simulink library "gnss_sdr_galileo_e1_tcp_connector_tracking_lib"  (Simulink 7.6)
settings: Solver=VariableStepDiscrete  StartTime=0.0  StopTime=10.0  RelTol=1e-3
undefined symbols (not defined in the file or in its folder): B_DLL, B_PLL, d_pdi_carr, d_pdi_code, k_DLL, k_PLL, magnitude, zeta_DLL, zeta_PLL
libraries: simulink x746, instrumentlib x2, dspindex x1
(part 1 of 5)
settings Model: Creator=David Pubill  LastModifiedBy=David Pubill

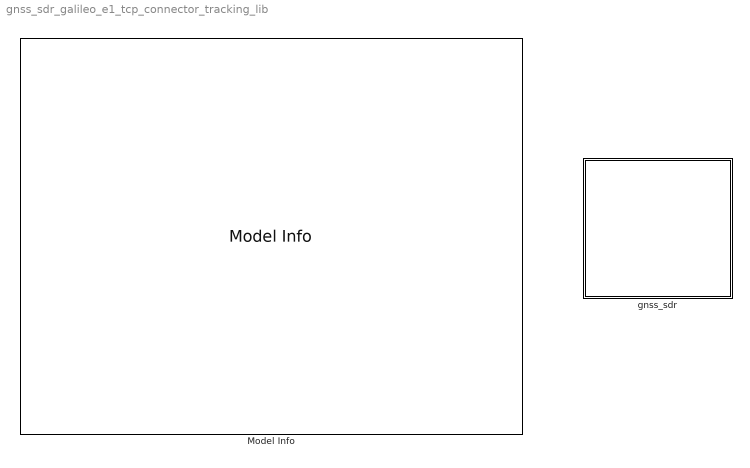
== system gnss_sdr_galileo_e1_tcp_connector_tracking_lib ==
  Model Info : simulink/Model-Wide Utilities/Model Info  SystemSampleTime=-1  InitialBlockCM=None  BlockCM=None  Frame=on  DisplayStringWithTags=|  HorizontalTextAlignment=Left  LeftAlignmentValue=0.02  SourceBlockDiagram=gnss_sdr_galileo_e1_tcp_connector_tracking_lib  TagMaxNumber=20
      | /*! 
      |   * \file gnss_sdr_galileo_e1_tcp_connector_tracking_lib.mdl
      |   * \brief  gnss_sdr_galileo_e1_tcp_connector_tracking Simulink library model. For 
      |   * further information, please check  the README_gnss_sdr_galileo_e1_tcp_connector_tracking.txt file.
      |   *
      |   * \author David Pubill, 2012. dpubill(at)cttc.es
      |   * -------------------------------------------------------------------------
      |   *
      |   * Copyright (C) 2010-2012  (see AUTHORS file for a list of contributors)
      |   *
      |   * GNSS-SDR is a software defined Global Navigation
      |   *          Satellite Systems receiver
      |   *
      |   * This file is part of GNSS-SDR.
      |   *
      |   * GNSS-SDR is free software: you can redistribute it and/or modify
      |   * it under the terms of the GNU General Public License as published by
      |   * the Free Software Foundation, either version 3 of the License, or
      |   * at your option) any later version.
      |   *
      |   * GNSS-SDR is distributed in the hope that it will be useful,
      |   * but WITHOUT ANY WARRANTY; without even the implied warranty of
      |   * MERCHANTABILITY or FITNESS FOR A PARTICULAR PURPOSE.  See the
      |   * GNU General Public License for more details.
      |   *
      |   * You should have received a copy of the GNU General Public License
      |   * along with GNSS-SDR. If not, see <http://www.gnu.org/licenses/>.
      |   *
      |   * -------------------------------------------------------------------------
      |   */
  gnss_sdr : Subsystem

== system gnss_sdr_galileo_e1_tcp_connector_tracking_lib/gnss_sdr ==
  gnss_sdr_galileo_e1_tcp_connector_tracking : Subsystem
  gnss_sdr_galileo_e1_tcp_connector_tracking_rx : Subsystem
  gnss_sdr_galileo_e1_tcp_connector_tracking_tx : Subsystem

== system gnss_sdr_galileo_e1_tcp_connector_tracking_lib/gnss_sdr/gnss_sdr_galileo_e1_tcp_connector_tracking ==
  control_id : Inport
  d_vE_I : Inport  Port=2
  d_vE_Q : Inport  Port=3
  d_E_I : Inport  Port=4
  d_E_Q : Inport  Port=5
  d_L_I : Inport  Port=6
  d_L_Q : Inport  Port=7
  d_vL_I : Inport  Port=8
  d_vL_Q : Inport  Port=9
  d_P_I : Inport  Port=10
  d_P_Q : Inport  Port=11
  d_acq_carrier_doppler_Hz : Inport  Port=12
  enable_tracking : Inport  Port=13
  Abs{,1..4} (5 alike) : Abs
  Carrier Tracking (PLL) : Subsystem
  Code Tracking (DLL) : Subsystem
  Data Type  Conversion1 : DataTypeConversion  OutDataTypeStr=single  SaturateOnIntegerOverflow=on  RndMeth=Zero
  Data Type  Conversion{2,5..9} (6 alike) : DataTypeConversion  OutDataTypeStr=double  SaturateOnIntegerOverflow=on  RndMeth=Zero
  Data Type  Conversion3 : DataTypeConversion  OutDataTypeStr=single  SaturateOnIntegerOverflow=on  RndMeth=Zero
  Data Type  Conversion4 : DataTypeConversion  OutDataTypeStr=single  SaturateOnIntegerOverflow=on  RndMeth=Zero
  Mux : Mux  Inputs=5
  Real-Imag to Complex{,1..4} (5 alike) : RealImagToComplex
  control_id_ : Outport
  code_nco : Outport  Port=2
  carr_nco : Outport  Port=3
  carrier_doppler_Hz : Outport  Port=4
  EPL Scope : Outport  Port=5
  wires:
  Data Type  Conversion8/1 -> Code Tracking (DLL)/4(vL), Abs3/1
  Data Type  Conversion7/1 -> Code Tracking (DLL)/1(vE), Abs4/1
  d_vL_Q/1 -> Real-Imag to Complex4/2
  d_vL_I/1 -> Real-Imag to Complex4/1
  Real-Imag to Complex4/1 -> Data Type  Conversion8/1
  d_vE_Q/1 -> Real-Imag to Complex3/2
  d_vE_I/1 -> Real-Imag to Complex3/1
  Real-Imag to Complex3/1 -> Data Type  Conversion7/1
  Mux/1 -> EPL Scope/1
  enable_tracking/1 -> Carrier Tracking (PLL)/3(enable_tracking), Code Tracking (DLL)/5(enable_tracking)
  Data Type  Conversion3/1 -> carrier_doppler_Hz/1
  d_acq_carrier_doppler_Hz/1 -> Data Type  Conversion9/1
  Data Type  Conversion6/1 -> Carrier Tracking (PLL)/1(P), Abs1/1
  Data Type  Conversion5/1 -> Abs/1, Code Tracking (DLL)/3(L)
  Data Type  Conversion2/1 -> Abs2/1, Code Tracking (DLL)/2(E)
  d_P_Q/1 -> Real-Imag to Complex2/2
  d_P_I/1 -> Real-Imag to Complex2/1
  d_L_Q/1 -> Real-Imag to Complex1/2
  d_L_I/1 -> Real-Imag to Complex1/1
  control_id/1 -> control_id_/1
  Data Type  Conversion4/1 -> carr_nco/1
  Data Type  Conversion1/1 -> code_nco/1
  d_E_Q/1 -> Real-Imag to Complex/2
  d_E_I/1 -> Real-Imag to Complex/1
  Real-Imag to Complex2/1 -> Data Type  Conversion6/1
  Real-Imag to Complex1/1 -> Data Type  Conversion5/1
  Carrier Tracking (PLL)/1(carr_nco) -> Data Type  Conversion4/1
  Real-Imag to Complex/1 -> Data Type  Conversion2/1
  Code Tracking (DLL)/1(code_nco) -> Data Type  Conversion1/1
  Carrier Tracking (PLL)/2(carrier_doppler_Hz) -> Data Type  Conversion3/1
  Abs4/1 -> Mux/1
  Abs2/1 -> Mux/2
  Abs1/1 -> Mux/3
  Abs/1 -> Mux/4
  Abs3/1 -> Mux/5
  Data Type  Conversion9/1 -> Carrier Tracking (PLL)/2(d_acq_carrier_doppler_Hz)

== system gnss_sdr_galileo_e1_tcp_connector_tracking_lib/gnss_sdr/gnss_sdr_galileo_e1_tcp_connector_tracking_rx ==
  Multiport Selector : dspindex/Multiport Selector  rowsOrCols=Rows  idxCellArray={1,2,3,4,5,6,7,8,9,10,11,12,13,14,15,16,17,18,19,20,21,22,23,24,25,26,27,28,29,30,31,32,33,34,35,36,37,38,39,40,41,42,43,44,45,46,47,48,49,50,51,52}  idxErrMode=Clip Index
  RX : instrumentlib/TCP//IP Receive  DialogController=instrumentcreatedialog  DialogControllerArgs=DataTag4  Host=84.88.61.86  Port=2070  DataSize=52  EnableBlockingMode=on  Timeout=5  SampleTime=-1  DataType=uint8  ByteOrder=BigEndian
  Subsystem : Subsystem
  Subsystem1 : Subsystem
  Subsystem10 : Subsystem  AncestorBlock=gnss_sdr_galileo_e1_tcp_connector_tracking_lib/gnss_sdr/gnss_sdr_galileo_e1_tcp_connector_tracking_rx/Subsystem1
  Subsystem11 : Subsystem  AncestorBlock=gnss_sdr_galileo_e1_tcp_connector_tracking_lib/gnss_sdr/gnss_sdr_galileo_e1_tcp_connector_tracking_rx/Subsystem2
  Subsystem12 : Subsystem  AncestorBlock=gnss_sdr_galileo_e1_tcp_connector_tracking_lib/gnss_sdr/gnss_sdr_galileo_e1_tcp_connector_tracking_rx/Subsystem3
  Subsystem2 : Subsystem
  Subsystem3 : Subsystem
  Subsystem4 : Subsystem
  Subsystem5 : Subsystem
  Subsystem6 : Subsystem
  Subsystem7 : Subsystem
  Subsystem8 : Subsystem
  Subsystem9 : Subsystem  AncestorBlock=gnss_sdr_galileo_e1_tcp_connector_tracking_lib/gnss_sdr/gnss_sdr_galileo_e1_tcp_connector_tracking_rx/Subsystem
  control_id : Outport
  d_vE_I : Outport  Port=2
  d_vE_Q : Outport  Port=3
  d_E_I : Outport  Port=4
  d_E_Q : Outport  Port=5
  d_L_I : Outport  Port=6
  d_L_Q : Outport  Port=7
  d_vL_I : Outport  Port=8
  d_vL_Q : Outport  Port=9
  d_P_I : Outport  Port=10
  d_P_Q : Outport  Port=11
  d_acq_carrier_doppler_Hz : Outport  Port=12
  enable_tracking : Outport  Port=13
  wires:
  Multiport Selector/52 -> Subsystem7/4(In4)
  Multiport Selector/51 -> Subsystem7/3(In3)
  Multiport Selector/50 -> Subsystem7/2(In2)
  Multiport Selector/49 -> Subsystem7/1(In1)
  Multiport Selector/48 -> Subsystem6/4(In4)
  Multiport Selector/47 -> Subsystem6/3(In3)
  Multiport Selector/46 -> Subsystem6/2(In2)
  Multiport Selector/45 -> Subsystem6/1(In1)
  Multiport Selector/44 -> Subsystem5/4(In4)
  Multiport Selector/43 -> Subsystem5/3(In3)
  Multiport Selector/42 -> Subsystem5/2(In2)
  Multiport Selector/41 -> Subsystem5/1(In1)
  Multiport Selector/40 -> Subsystem4/4(In4)
  Multiport Selector/39 -> Subsystem4/3(In3)
  Multiport Selector/38 -> Subsystem4/2(In2)
  Multiport Selector/37 -> Subsystem4/1(In1)
  Multiport Selector/36 -> Subsystem12/4(In4)
  Multiport Selector/35 -> Subsystem12/3(In3)
  Multiport Selector/34 -> Subsystem12/2(In2)
  Multiport Selector/33 -> Subsystem12/1(In1)
  Multiport Selector/32 -> Subsystem11/4(In4)
  Multiport Selector/31 -> Subsystem11/3(In3)
  Multiport Selector/30 -> Subsystem11/2(In2)
  Multiport Selector/29 -> Subsystem11/1(In1)
  Multiport Selector/28 -> Subsystem3/4(In4)
  Multiport Selector/27 -> Subsystem3/3(In3)
  Multiport Selector/26 -> Subsystem3/2(In2)
  Multiport Selector/25 -> Subsystem3/1(In1)
  Multiport Selector/24 -> Subsystem2/4(In4)
  Multiport Selector/23 -> Subsystem2/3(In3)
  Multiport Selector/22 -> Subsystem2/2(In2)
  Multiport Selector/21 -> Subsystem2/1(In1)
  Multiport Selector/20 -> Subsystem1/4(In4)
  Multiport Selector/19 -> Subsystem1/3(In3)
  Multiport Selector/18 -> Subsystem1/2(In2)
  Multiport Selector/17 -> Subsystem1/1(In1)
  Multiport Selector/16 -> Subsystem/4(In4)
  Multiport Selector/15 -> Subsystem/3(In3)
  Multiport Selector/14 -> Subsystem/2(In2)
  Multiport Selector/13 -> Subsystem/1(In1)
  Multiport Selector/12 -> Subsystem10/4(In4)
  Multiport Selector/11 -> Subsystem10/3(In3)
  Multiport Selector/10 -> Subsystem10/2(In2)
  Multiport Selector/9 -> Subsystem10/1(In1)
  Multiport Selector/8 -> Subsystem9/4(In4)
  Multiport Selector/7 -> Subsystem9/3(In3)
  Multiport Selector/6 -> Subsystem9/2(In2)
  Multiport Selector/5 -> Subsystem9/1(In1)
  Multiport Selector/4 -> Subsystem8/4(In4)
  Multiport Selector/3 -> Subsystem8/3(In3)
  Multiport Selector/2 -> Subsystem8/2(In2)
  Multiport Selector/1 -> Subsystem8/1(In1)
  Subsystem11/1(d_vL_I) -> d_vL_I/1
  Subsystem12/1(d_vL_Q) -> d_vL_Q/1
  Subsystem9/1(d_vE_I) -> d_vE_I/1
  Subsystem10/1(d_vE_Q) -> d_vE_Q/1
  Subsystem7/1(enable_tracking) -> enable_tracking/1
  Subsystem6/1(d_acq_carrier_doppler_Hz) -> d_acq_carrier_doppler_Hz/1
  Subsystem5/1(d_P_Q) -> d_P_Q/1
  Subsystem8/1(control_id) -> control_id/1
  Subsystem/1(d_E_I) -> d_E_I/1
  Subsystem1/1(d_E_Q) -> d_E_Q/1
  Subsystem2/1(d_L_I) -> d_L_I/1
  Subsystem3/1(d_L_Q) -> d_L_Q/1
  Subsystem4/1(d_P_I) -> d_P_I/1
  RX/1 -> Multiport Selector/1

== system gnss_sdr_galileo_e1_tcp_connector_tracking_lib/gnss_sdr/gnss_sdr_galileo_e1_tcp_connector_tracking_tx ==
  control_id : Inport
  code_nco : Inport  Port=2
  carr_nco : Inport  Port=3
  carrier_doppler_Hz : Inport  Port=4
  TX : instrumentlib/TCP//IP Send  DialogController=instrumentcreatedialog  DialogControllerArgs=DataTag5  Host=84.88.61.86  Port=2070  EnableBlockingMode=on  Timeout=5  ByteOrder=LittleEndian
  Vector Concatenate1 : Concatenate  NumInputs=4  Mode=Vector
  wires:
  carrier_doppler_Hz/1 -> Vector Concatenate1/4
  Vector Concatenate1/1 -> TX/1
  control_id/1 -> Vector Concatenate1/1
  code_nco/1 -> Vector Concatenate1/2
  carr_nco/1 -> Vector Concatenate1/3

== system gnss_sdr_galileo_e1_tcp_connector_tracking_lib/gnss_sdr/gnss_sdr_galileo_e1_tcp_connector_tracking/Carrier Tracking (PLL) ==
  P : Inport
  d_acq_carrier_doppler_Hz : Inport  Port=2
  enable_tracking : Inport  Port=3
  Constant : Constant  Value=0  SampleTime=-1
  PLL Filter : Subsystem
  PLL discriminator : Subsystem  AncestorBlock=|
      | gnss_sdr_tcp_connector_tracking_lib/gnss_sdr/gnss_sdr_tcp_connector_tracking/Carrier Tracking 
      | (PLL)/atan2(Q,I)1/PLL Costas loop two quadrant arctan discriminator
  Subtract : Sum
  Switch : Switch  Threshold=1
  "[rad/s] to [Hz]" : Gain  Gain=1/(2*pi)
  carr_nco : Outport
  carrier_doppler_Hz : Outport  Port=2
  wires:
  PLL discriminator/1(carr_error) -> "[rad/s] to [Hz]"/1
  P/1 -> PLL discriminator/1(P)
  enable_tracking/1 -> Switch/2, PLL Filter/2(enable_tracking)
  PLL Filter/1(carr_nco) -> Subtract/1, Switch/1
  d_acq_carrier_doppler_Hz/1 -> Subtract/2
  Subtract/1 -> carrier_doppler_Hz/1
  Switch/1 -> carr_nco/1
  Constant/1 -> Switch/3
  "[rad/s] to [Hz]"/1 -> PLL Filter/1(carr_error)

== system gnss_sdr_galileo_e1_tcp_connector_tracking_lib/gnss_sdr/gnss_sdr_galileo_e1_tcp_connector_tracking/Code Tracking (DLL) ==
  vE : Inport
  E : Inport  Port=2
  L : Inport  Port=3
  vL : Inport  Port=4
  enable_tracking : Inport  Port=5
  DLL Filter : Subsystem
  DLL discriminator : Subsystem
  code_nco : Outport
  wires:
  vL/1 -> DLL discriminator/4(vL)
  vE/1 -> DLL discriminator/1(vE)
  E/1 -> DLL discriminator/2(E)
  L/1 -> DLL discriminator/3(L)
  DLL Filter/1(code_nco) -> code_nco/1
  DLL discriminator/1(code_error) -> DLL Filter/1(code_error)
  enable_tracking/1 -> DLL Filter/2(enable_tracking)

== system gnss_sdr_galileo_e1_tcp_connector_tracking_lib/gnss_sdr/gnss_sdr_galileo_e1_tcp_connector_tracking_rx/Subsystem ==
  In1 : Inport
  In2 : Inport  Port=2
  In3 : Inport  Port=3
  In4 : Inport  Port=4
  Data Type  Conversion{1..5} (5 alike) : DataTypeConversion  OutDataTypeStr=single  SaturateOnIntegerOverflow=on  RndMeth=Zero
  hex2float : Subsystem
  d_E_I : Outport  OutputWhenDisabled=reset  InitialOutput=0
  wires:
  In1/1 -> Data Type  Conversion3/1
  In2/1 -> Data Type  Conversion2/1
  In3/1 -> Data Type  Conversion1/1
  In4/1 -> Data Type  Conversion4/1
  Data Type  Conversion3/1 -> hex2float/4(In4)
  Data Type  Conversion2/1 -> hex2float/3(In3)
  Data Type  Conversion1/1 -> hex2float/2(In2)
  Data Type  Conversion4/1 -> hex2float/1(In1)
  hex2float/1(Out1) -> Data Type  Conversion5/1
  Data Type  Conversion5/1 -> d_E_I/1

== system gnss_sdr_galileo_e1_tcp_connector_tracking_lib/gnss_sdr/gnss_sdr_galileo_e1_tcp_connector_tracking_rx/Subsystem1 ==
  In1 : Inport
  In2 : Inport  Port=2
  In3 : Inport  Port=3
  In4 : Inport  Port=4
  Data Type  Conversion{1..5} (5 alike) : DataTypeConversion  OutDataTypeStr=single  SaturateOnIntegerOverflow=on  RndMeth=Zero
  hex2float : Subsystem
  d_E_Q : Outport  OutputWhenDisabled=reset  InitialOutput=0
  wires:
  Data Type  Conversion5/1 -> d_E_Q/1
  hex2float/1(Out1) -> Data Type  Conversion5/1
  Data Type  Conversion4/1 -> hex2float/1(In1)
  Data Type  Conversion1/1 -> hex2float/2(In2)
  Data Type  Conversion2/1 -> hex2float/3(In3)
  Data Type  Conversion3/1 -> hex2float/4(In4)
  In4/1 -> Data Type  Conversion4/1
  In3/1 -> Data Type  Conversion1/1
  In2/1 -> Data Type  Conversion2/1
  In1/1 -> Data Type  Conversion3/1

== system gnss_sdr_galileo_e1_tcp_connector_tracking_lib/gnss_sdr/gnss_sdr_galileo_e1_tcp_connector_tracking_rx/Subsystem10 ==
  In1 : Inport
  In2 : Inport  Port=2
  In3 : Inport  Port=3
  In4 : Inport  Port=4
  Data Type  Conversion{1..5} (5 alike) : DataTypeConversion  OutDataTypeStr=single  SaturateOnIntegerOverflow=on  RndMeth=Zero
  hex2float : Subsystem
  d_vE_Q : Outport  OutputWhenDisabled=reset  InitialOutput=0
  wires:
  Data Type  Conversion5/1 -> d_vE_Q/1
  hex2float/1(Out1) -> Data Type  Conversion5/1
  Data Type  Conversion4/1 -> hex2float/1(In1)
  Data Type  Conversion1/1 -> hex2float/2(In2)
  Data Type  Conversion2/1 -> hex2float/3(In3)
  Data Type  Conversion3/1 -> hex2float/4(In4)
  In4/1 -> Data Type  Conversion4/1
  In3/1 -> Data Type  Conversion1/1
  In2/1 -> Data Type  Conversion2/1
  In1/1 -> Data Type  Conversion3/1

== system gnss_sdr_galileo_e1_tcp_connector_tracking_lib/gnss_sdr/gnss_sdr_galileo_e1_tcp_connector_tracking_rx/Subsystem11 ==
  In1 : Inport
  In2 : Inport  Port=2
  In3 : Inport  Port=3
  In4 : Inport  Port=4
  Data Type  Conversion{1..5} (5 alike) : DataTypeConversion  OutDataTypeStr=single  SaturateOnIntegerOverflow=on  RndMeth=Zero
  hex2float : Subsystem
  d_vL_I : Outport  OutputWhenDisabled=reset  InitialOutput=0
  wires:
  In1/1 -> Data Type  Conversion3/1
  In2/1 -> Data Type  Conversion2/1
  In3/1 -> Data Type  Conversion1/1
  In4/1 -> Data Type  Conversion4/1
  Data Type  Conversion3/1 -> hex2float/4(In4)
  Data Type  Conversion2/1 -> hex2float/3(In3)
  Data Type  Conversion1/1 -> hex2float/2(In2)
  Data Type  Conversion4/1 -> hex2float/1(In1)
  hex2float/1(Out1) -> Data Type  Conversion5/1
  Data Type  Conversion5/1 -> d_vL_I/1

== system gnss_sdr_galileo_e1_tcp_connector_tracking_lib/gnss_sdr/gnss_sdr_galileo_e1_tcp_connector_tracking_rx/Subsystem12 ==
  In1 : Inport
  In2 : Inport  Port=2
  In3 : Inport  Port=3
  In4 : Inport  Port=4
  Data Type  Conversion{1..5} (5 alike) : DataTypeConversion  OutDataTypeStr=single  SaturateOnIntegerOverflow=on  RndMeth=Zero
  hex2float : Subsystem
  d_vL_Q : Outport  OutputWhenDisabled=reset  InitialOutput=0
  wires:
  Data Type  Conversion5/1 -> d_vL_Q/1
  hex2float/1(Out1) -> Data Type  Conversion5/1
  Data Type  Conversion4/1 -> hex2float/1(In1)
  Data Type  Conversion1/1 -> hex2float/2(In2)
  Data Type  Conversion2/1 -> hex2float/3(In3)
  Data Type  Conversion3/1 -> hex2float/4(In4)
  In4/1 -> Data Type  Conversion4/1
  In3/1 -> Data Type  Conversion1/1
  In2/1 -> Data Type  Conversion2/1
  In1/1 -> Data Type  Conversion3/1

== system gnss_sdr_galileo_e1_tcp_connector_tracking_lib/gnss_sdr/gnss_sdr_galileo_e1_tcp_connector_tracking_rx/Subsystem2 ==
  In1 : Inport
  In2 : Inport  Port=2
  In3 : Inport  Port=3
  In4 : Inport  Port=4
  Data Type  Conversion{1..5} (5 alike) : DataTypeConversion  OutDataTypeStr=single  SaturateOnIntegerOverflow=on  RndMeth=Zero
  hex2float : Subsystem
  d_L_I : Outport  OutputWhenDisabled=reset  InitialOutput=0
  wires:
  In1/1 -> Data Type  Conversion3/1
  In2/1 -> Data Type  Conversion2/1
  In3/1 -> Data Type  Conversion1/1
  In4/1 -> Data Type  Conversion4/1
  Data Type  Conversion3/1 -> hex2float/4(In4)
  Data Type  Conversion2/1 -> hex2float/3(In3)
  Data Type  Conversion1/1 -> hex2float/2(In2)
  Data Type  Conversion4/1 -> hex2float/1(In1)
  hex2float/1(Out1) -> Data Type  Conversion5/1
  Data Type  Conversion5/1 -> d_L_I/1

== system gnss_sdr_galileo_e1_tcp_connector_tracking_lib/gnss_sdr/gnss_sdr_galileo_e1_tcp_connector_tracking_rx/Subsystem3 ==
  In1 : Inport
  In2 : Inport  Port=2
  In3 : Inport  Port=3
  In4 : Inport  Port=4
  Data Type  Conversion{1..5} (5 alike) : DataTypeConversion  OutDataTypeStr=single  SaturateOnIntegerOverflow=on  RndMeth=Zero
  hex2float : Subsystem
  d_L_Q : Outport  OutputWhenDisabled=reset  InitialOutput=0
  wires:
  Data Type  Conversion5/1 -> d_L_Q/1
  hex2float/1(Out1) -> Data Type  Conversion5/1
  Data Type  Conversion4/1 -> hex2float/1(In1)
  Data Type  Conversion1/1 -> hex2float/2(In2)
  Data Type  Conversion2/1 -> hex2float/3(In3)
  Data Type  Conversion3/1 -> hex2float/4(In4)
  In4/1 -> Data Type  Conversion4/1
  In3/1 -> Data Type  Conversion1/1
  In2/1 -> Data Type  Conversion2/1
  In1/1 -> Data Type  Conversion3/1

== system gnss_sdr_galileo_e1_tcp_connector_tracking_lib/gnss_sdr/gnss_sdr_galileo_e1_tcp_connector_tracking_rx/Subsystem4 ==
  In1 : Inport
  In2 : Inport  Port=2
  In3 : Inport  Port=3
  In4 : Inport  Port=4
  Data Type  Conversion{1..5} (5 alike) : DataTypeConversion  OutDataTypeStr=single  SaturateOnIntegerOverflow=on  RndMeth=Zero
  hex2float : Subsystem
  d_P_I : Outport  OutputWhenDisabled=reset  InitialOutput=0
  wires:
  Data Type  Conversion5/1 -> d_P_I/1
  hex2float/1(Out1) -> Data Type  Conversion5/1
  Data Type  Conversion4/1 -> hex2float/1(In1)
  Data Type  Conversion1/1 -> hex2float/2(In2)
  Data Type  Conversion2/1 -> hex2float/3(In3)
  Data Type  Conversion3/1 -> hex2float/4(In4)
  In4/1 -> Data Type  Conversion4/1
  In3/1 -> Data Type  Conversion1/1
  In2/1 -> Data Type  Conversion2/1
  In1/1 -> Data Type  Conversion3/1

== system gnss_sdr_galileo_e1_tcp_connector_tracking_lib/gnss_sdr/gnss_sdr_galileo_e1_tcp_connector_tracking_rx/Subsystem5 ==
  In1 : Inport
  In2 : Inport  Port=2
  In3 : Inport  Port=3
  In4 : Inport  Port=4
  Data Type  Conversion{1..5} (5 alike) : DataTypeConversion  OutDataTypeStr=single  SaturateOnIntegerOverflow=on  RndMeth=Zero
  hex2float : Subsystem
  d_P_Q : Outport  OutputWhenDisabled=reset  InitialOutput=0
  wires:
  In1/1 -> Data Type  Conversion3/1
  In2/1 -> Data Type  Conversion2/1
  In3/1 -> Data Type  Conversion1/1
  In4/1 -> Data Type  Conversion4/1
  Data Type  Conversion3/1 -> hex2float/4(In4)
  Data Type  Conversion2/1 -> hex2float/3(In3)
  Data Type  Conversion1/1 -> hex2float/2(In2)
  Data Type  Conversion4/1 -> hex2float/1(In1)
  hex2float/1(Out1) -> Data Type  Conversion5/1
  Data Type  Conversion5/1 -> d_P_Q/1

== system gnss_sdr_galileo_e1_tcp_connector_tracking_lib/gnss_sdr/gnss_sdr_galileo_e1_tcp_connector_tracking_rx/Subsystem6 ==
  In1 : Inport
  In2 : Inport  Port=2
  In3 : Inport  Port=3
  In4 : Inport  Port=4
  Data Type  Conversion{1..5} (5 alike) : DataTypeConversion  OutDataTypeStr=single  SaturateOnIntegerOverflow=on  RndMeth=Zero
  hex2float : Subsystem
  d_acq_carrier_doppler_Hz : Outport  OutputWhenDisabled=reset  InitialOutput=0
  wires:
  Data Type  Conversion5/1 -> d_acq_carrier_doppler_Hz/1
  hex2float/1(Out1) -> Data Type  Conversion5/1
  Data Type  Conversion4/1 -> hex2float/1(In1)
  Data Type  Conversion1/1 -> hex2float/2(In2)
  Data Type  Conversion2/1 -> hex2float/3(In3)
  Data Type  Conversion3/1 -> hex2float/4(In4)
  In4/1 -> Data Type  Conversion4/1
  In3/1 -> Data Type  Conversion1/1
  In2/1 -> Data Type  Conversion2/1
  In1/1 -> Data Type  Conversion3/1

== system gnss_sdr_galileo_e1_tcp_connector_tracking_lib/gnss_sdr/gnss_sdr_galileo_e1_tcp_connector_tracking_rx/Subsystem7 ==
  In1 : Inport
  In2 : Inport  Port=2
  In3 : Inport  Port=3
  In4 : Inport  Port=4
  Data Type  Conversion{1..5} (5 alike) : DataTypeConversion  OutDataTypeStr=single  SaturateOnIntegerOverflow=on  RndMeth=Zero
  hex2float : Subsystem
  enable_tracking : Outport  OutputWhenDisabled=reset  InitialOutput=0
  wires:
  In1/1 -> Data Type  Conversion3/1
  In2/1 -> Data Type  Conversion2/1
  In3/1 -> Data Type  Conversion1/1
  In4/1 -> Data Type  Conversion4/1
  Data Type  Conversion3/1 -> hex2float/4(In4)
  Data Type  Conversion2/1 -> hex2float/3(In3)
  Data Type  Conversion1/1 -> hex2float/2(In2)
  Data Type  Conversion4/1 -> hex2float/1(In1)
  hex2float/1(Out1) -> Data Type  Conversion5/1
  Data Type  Conversion5/1 -> enable_tracking/1

== system gnss_sdr_galileo_e1_tcp_connector_tracking_lib/gnss_sdr/gnss_sdr_galileo_e1_tcp_connector_tracking_rx/Subsystem8 ==
  In1 : Inport
  In2 : Inport  Port=2
  In3 : Inport  Port=3
  In4 : Inport  Port=4
  Data Type  Conversion{1..5} (5 alike) : DataTypeConversion  OutDataTypeStr=single  SaturateOnIntegerOverflow=on  RndMeth=Zero
  hex2float : Subsystem
  control_id : Outport  OutputWhenDisabled=reset  InitialOutput=0
  wires:
  In1/1 -> Data Type  Conversion3/1
  In2/1 -> Data Type  Conversion2/1
  In3/1 -> Data Type  Conversion1/1
  In4/1 -> Data Type  Conversion4/1
  Data Type  Conversion3/1 -> hex2float/4(In4)
  Data Type  Conversion2/1 -> hex2float/3(In3)
  Data Type  Conversion1/1 -> hex2float/2(In2)
  Data Type  Conversion4/1 -> hex2float/1(In1)
  hex2float/1(Out1) -> Data Type  Conversion5/1
  Data Type  Conversion5/1 -> control_id/1

== system gnss_sdr_galileo_e1_tcp_connector_tracking_lib/gnss_sdr/gnss_sdr_galileo_e1_tcp_connector_tracking_rx/Subsystem9 ==
  In1 : Inport
  In2 : Inport  Port=2
  In3 : Inport  Port=3
  In4 : Inport  Port=4
  Data Type  Conversion{1..5} (5 alike) : DataTypeConversion  OutDataTypeStr=single  SaturateOnIntegerOverflow=on  RndMeth=Zero
  hex2float : Subsystem
  d_vE_I : Outport  OutputWhenDisabled=reset  InitialOutput=0
  wires:
  In1/1 -> Data Type  Conversion3/1
  In2/1 -> Data Type  Conversion2/1
  In3/1 -> Data Type  Conversion1/1
  In4/1 -> Data Type  Conversion4/1
  Data Type  Conversion3/1 -> hex2float/4(In4)
  Data Type  Conversion2/1 -> hex2float/3(In3)
  Data Type  Conversion1/1 -> hex2float/2(In2)
  Data Type  Conversion4/1 -> hex2float/1(In1)
  hex2float/1(Out1) -> Data Type  Conversion5/1
  Data Type  Conversion5/1 -> d_vE_I/1

== system gnss_sdr_galileo_e1_tcp_connector_tracking_lib/gnss_sdr/gnss_sdr_galileo_e1_tcp_connector_tracking/Carrier Tracking (PLL)/PLL Filter ==
  carr_error : Inport
  enable_tracking : Inport  Port=2
  2*zeta : Constant  Value=2*zeta_PLL  SampleTime=-1
  Add1 : Sum  Inputs=+++
  Constant4 : Constant  Value=0  SampleTime=-1
  Constant5 : Constant  Value=0  SampleTime=-1
  Constant6 : Constant  Value=0  SampleTime=-1
  Delay1 : simulink/Discrete/Integer Delay  NumDelays=1  InputProcessing=Inherited  vinit=0.0  samptime=-1
  Delay3 : simulink/Discrete/Integer Delay  NumDelays=1  InputProcessing=Inherited  vinit=0.0  samptime=-1
  Divide{4..7} (4 alike) : Product  Inputs=*/
  Product4 : Product  RndMeth=Zero
  Product5 : Product  RndMeth=Zero
  Product6 : Product  RndMeth=Zero
  Subtract1 : Sum  Inputs=+-
  Switch4 : Switch  Threshold=1
  Switch5 : Switch  Threshold=1
  Switch6 : Switch  Threshold=1
  Wn : Gain  Gain=(8*zeta_PLL)/(1+(4*(zeta_PLL)^2))
  d_pdi_carr : Constant  Value=d_pdi_carr  SampleTime=-1
  k : Constant  Value=k_PLL  SampleTime=-1
  lbw : Constant  Value=B_PLL  SampleTime=-1
  carr_nco : Outport
  wires:
  d_pdi_carr/1 -> Divide7/1
  Divide7/1 -> Product6/2
  Add1/1 -> carr_nco/1, Delay1/1
  Product5/1 -> Add1/1
  Divide6/1 -> Product5/2
  carr_error/1 -> Product6/1, Subtract1/1, Switch4/1
  Divide5/1 -> Divide6/1  "Tau2"
  2*zeta/1 -> Divide5/1
  Product4/1 -> Divide4/2
  k/1 -> Divide4/1
  Divide4/1 -> Divide7/2, Divide6/2  "Tau1"
  lbw/1 -> Wn/1
  Wn/1 -> Product4/2, Product4/1, Divide5/2
  Delay1/1 -> Add1/3
  Subtract1/1 -> Switch6/1
  Switch6/1 -> Product5/1
  Product6/1 -> Switch5/1
  Switch5/1 -> Add1/2
  Constant5/1 -> Switch5/3
  Delay3/1 -> Subtract1/2
  Constant6/1 -> Switch4/3
  enable_tracking/1 -> Switch6/2, Switch4/2, Switch5/2
  Constant4/1 -> Switch6/3
  Switch4/1 -> Delay3/1

== system gnss_sdr_galileo_e1_tcp_connector_tracking_lib/gnss_sdr/gnss_sdr_galileo_e1_tcp_connector_tracking/Carrier Tracking (PLL)/PLL discriminator ==
  P : Inport
  Abs : Abs
  Complex to Real-Imag : ComplexToRealImag
  Constant : Constant  Value=0  SampleTime=-1
  Divide : Product  Inputs=*/
  Switch : Switch  Criteria=u2 > Threshold
  Trigonometric Function : Trigonometry  Operator=atan
  carr_error : Outport
  wires:
  Abs/1 -> Switch/2
  Trigonometric Function/1 -> Switch/1
  Switch/1 -> carr_error/1
  Constant/1 -> Switch/3
  Complex to Real-Imag/2 -> Divide/1
  Complex to Real-Imag/1 -> Divide/2, Abs/1
  Divide/1 -> Trigonometric Function/1
  P/1 -> Complex to Real-Imag/1

== system gnss_sdr_galileo_e1_tcp_connector_tracking_lib/gnss_sdr/gnss_sdr_galileo_e1_tcp_connector_tracking/Code Tracking (DLL)/DLL Filter ==
  code_error : Inport
  enable_tracking : Inport  Port=2
  2*zeta : Constant  Value=2*zeta_DLL  SampleTime=-1
  Add : Sum  Inputs=+++
  Constant : Constant  Value=0  SampleTime=-1
  Constant2 : Constant  Value=0  SampleTime=-1
  Constant3 : Constant  Value=0  SampleTime=-1
  Delay : simulink/Discrete/Integer Delay  NumDelays=1  InputProcessing=Inherited  vinit=0.0  samptime=-1
  Delay2 : simulink/Discrete/Integer Delay  NumDelays=1  InputProcessing=Inherited  vinit=0.0  samptime=-1
  Divide{,2,4..5} (4 alike) : Product  Inputs=*/
  Product1 : Product  RndMeth=Zero
  Product2 : Product  RndMeth=Zero
  Product3 : Product  RndMeth=Zero
  Subtract : Sum  Inputs=+-
  Switch1 : Switch  Threshold=1
  Switch2 : Switch  Threshold=1
  Switch4 : Switch  Threshold=1
  Wn : Gain  Gain=(8*zeta_DLL)/(1+(4*(zeta_DLL)^2))
  d_pdi_code : Constant  Value=d_pdi_code  SampleTime=-1
  k : Constant  Value=k_DLL  SampleTime=-1
  lbw : Constant  Value=B_DLL  SampleTime=-1
  code_nco : Outport
  wires:
  d_pdi_code/1 -> Divide5/1
  Divide5/1 -> Product3/2
  Add/1 -> code_nco/1, Delay/1
  Product2/1 -> Add/1
  Divide4/1 -> Product2/2
  code_error/1 -> Product3/1, Subtract/1, Switch1/1
  Divide2/1 -> Divide4/1  "Tau2"
  2*zeta/1 -> Divide2/1
  Product1/1 -> Divide/2
  k/1 -> Divide/1
  Divide/1 -> Divide5/2, Divide4/2  "Tau1"
  lbw/1 -> Wn/1
  Wn/1 -> Product1/2, Product1/1, Divide2/2
  Delay/1 -> Add/3
  Subtract/1 -> Switch4/1
  Switch4/1 -> Product2/1
  Product3/1 -> Switch2/1
  Switch2/1 -> Add/2
  Constant2/1 -> Switch2/3
  Delay2/1 -> Subtract/2
  Constant3/1 -> Switch1/3
  enable_tracking/1 -> Switch4/2, Switch1/2, Switch2/2
  Constant/1 -> Switch4/3
  Switch1/1 -> Delay2/1

== system gnss_sdr_galileo_e1_tcp_connector_tracking_lib/gnss_sdr/gnss_sdr_galileo_e1_tcp_connector_tracking/Code Tracking (DLL)/DLL discriminator ==
  vE : Inport
  E : Inport  Port=2
  L : Inport  Port=3
  vL : Inport  Port=4
  E power : Math  Operator=magnitude^2  SaturateOnIntegerOverflow=on
  L power : Math  Operator=magnitude^2  SaturateOnIntegerOverflow=on
  Sqrt : Sqrt  SaturateOnIntegerOverflow=on
  Sqrt1 : Sqrt  SaturateOnIntegerOverflow=on
  Sum : Sum  Inputs=+|-  SaturateOnIntegerOverflow=on
  Sum1 : Sum  Inputs=+|+  SaturateOnIntegerOverflow=on
  Sum2 : Sum  Inputs=+|+  SaturateOnIntegerOverflow=on
  Sum3 : Sum  Inputs=+|+  SaturateOnIntegerOverflow=on
  vE Normalisation : Product  Inputs=*/  SaturateOnIntegerOverflow=on  OutDataTypeStr=Inherit: Same as first input
  vE power : Math  Operator=magnitude^2  SaturateOnIntegerOverflow=on
  vL power : Math  Operator=magnitude^2  SaturateOnIntegerOverflow=on
  code_error : Outport
  wires:
  vL power/1 -> Sum3/2
  Sum3/1 -> Sqrt1/1
  L power/1 -> Sum3/1
  E power/1 -> Sum2/2
  Sum2/1 -> Sqrt/1
  vE Normalisation/1 -> code_error/1
  Sum1/1 -> vE Normalisation/2
  Sum/1 -> vE Normalisation/1
  vL/1 -> vL power/1
  vE/1 -> vE power/1
  vE power/1 -> Sum2/1
  L/1 -> L power/1
  E/1 -> E power/1
  Sqrt/1 -> Sum1/1, Sum/1
  Sqrt1/1 -> Sum1/2, Sum/2

== system gnss_sdr_galileo_e1_tcp_connector_tracking_lib/gnss_sdr/gnss_sdr_galileo_e1_tcp_connector_tracking_rx/Subsystem/hex2float ==
  In1 : Inport
  In2 : Inport  Port=2
  In3 : Inport  Port=3
  In4 : Inport  Port=4
  Bitwise Operator : simulink/Logic and Bit Operations/Bitwise Operator  logicop=AND  UseBitMask=on  BitMask=bin2dec('01111111')  BitMaskRealWorld=Stored Integer
  Bitwise Operator1 : simulink/Logic and Bit Operations/Bitwise Operator  logicop=AND  UseBitMask=on  BitMask=bin2dec('10000000')  BitMaskRealWorld=Stored Integer
  Bitwise Operator2 : simulink/Logic and Bit Operations/Bitwise Operator  logicop=AND  UseBitMask=on  BitMask=bin2dec('10000000')  BitMaskRealWorld=Stored Integer
  Bitwise Operator3 : simulink/Logic and Bit Operations/Bitwise Operator  logicop=AND  UseBitMask=on  BitMask=bin2dec('01111111')  BitMaskRealWorld=Stored Integer
  Constant4 : Constant  Value=127
  Constant5 : Constant  Value=8388608
  Constant7 : Constant  Value=-1
  Data Type Conversion : DataTypeConversion  OutDataTypeStr=uint8
  Data Type Conversion1 : DataTypeConversion  OutDataTypeStr=uint8
  Data Type Conversion{2..5} (4 alike) : DataTypeConversion  OutDataTypeStr=uint32
  Data Type Conversion7 : DataTypeConversion  OutDataTypeStr=double
  Display3 : Display
      settings: Format=binary (Stored Integer)
  Display4 : Display
      settings: Format=binary (Stored Integer)
  Exponent : Display
      settings: Format=binary (Stored Integer)
  Mantissa : Display
      settings: Format=binary (Stored Integer)
  Math Function : Math  Operator=pow  SaturateOnIntegerOverflow=on
  Product : Product  RndMeth=Zero
  Shift Arithmetic : simulink/Logic and Bit Operations/Shift Arithmetic  SystemSampleTime=-1  nBitShiftRight=-1  nBinPtShiftRight=0
  Shift Arithmetic1 : simulink/Logic and Bit Operations/Shift Arithmetic  SystemSampleTime=-1  nBitShiftRight=7  nBinPtShiftRight=0
  Shift Arithmetic2 : simulink/Logic and Bit Operations/Shift Arithmetic  SystemSampleTime=-1  nBitShiftRight=7  nBinPtShiftRight=0
  Shift Arithmetic3 : simulink/Logic and Bit Operations/Shift Arithmetic  SystemSampleTime=-1  nBitShiftRight=-16  nBinPtShiftRight=0
  Shift Arithmetic4 : simulink/Logic and Bit Operations/Shift Arithmetic  SystemSampleTime=-1  nBitShiftRight=-8  nBinPtShiftRight=0
  Sign : Display
      settings: Format=binary (Stored Integer)
  Subsystem : Subsystem
  Sum : Sum  Inputs=|++
  Sum1 : Sum  Inputs=|+++|
  Sum2 : Sum  Inputs=|+-
  Sum3 : Sum  Inputs=|++
  Out1 : Outport
  wires:
  In4/1 -> Data Type Conversion4/1
  In3/1 -> Data Type Conversion3/1
  Product/1 -> Out1/1
  In1/1 -> Data Type Conversion/1
  Math Function/1 -> Product/1
  Data Type Conversion7/1 -> Math Function/2
  Constant7/1 -> Math Function/1
  Subsystem/1(Out1) -> Product/2
  Data Type Conversion5/1 -> Sum3/2
  Constant5/1 -> Data Type Conversion5/1
  Sum3/1 -> Subsystem/2(In2)
  Sum2/1 -> Subsystem/1(In1)
  Constant4/1 -> Sum2/2
  Sum1/1 -> Sum3/1, Mantissa/1
  Data Type Conversion4/1 -> Sum1/3
  Shift Arithmetic4/1 -> Sum1/2
  Data Type Conversion3/1 -> Shift Arithmetic4/1
  Shift Arithmetic3/1 -> Sum1/1
  Data Type Conversion2/1 -> Bitwise Operator3/1
  Bitwise Operator3/1 -> Shift Arithmetic3/1
  Shift Arithmetic2/1 -> Data Type Conversion7/1, Sign/1
  Bitwise Operator2/1 -> Shift Arithmetic2/1
  Sum/1 -> Sum2/1, Exponent/1
  Shift Arithmetic1/1 -> Sum/2
  Bitwise Operator1/1 -> Shift Arithmetic1/1
  Shift Arithmetic/1 -> Sum/1, Display4/1
  Data Type Conversion1/1 -> Bitwise Operator1/1
  In2/1 -> Data Type Conversion1/1, Data Type Conversion2/1
  Data Type Conversion/1 -> Bitwise Operator2/1, Bitwise Operator/1
  Bitwise Operator/1 -> Shift Arithmetic/1, Display3/1

== system gnss_sdr_galileo_e1_tcp_connector_tracking_lib/gnss_sdr/gnss_sdr_galileo_e1_tcp_connector_tracking_rx/Subsystem1/hex2float ==
  In1 : Inport
  In2 : Inport  Port=2
  In3 : Inport  Port=3
  In4 : Inport  Port=4
  Bitwise Operator : simulink/Logic and Bit Operations/Bitwise Operator  logicop=AND  UseBitMask=on  BitMask=bin2dec('01111111')  BitMaskRealWorld=Stored Integer
  Bitwise Operator1 : simulink/Logic and Bit Operations/Bitwise Operator  logicop=AND  UseBitMask=on  BitMask=bin2dec('10000000')  BitMaskRealWorld=Stored Integer
  Bitwise Operator2 : simulink/Logic and Bit Operations/Bitwise Operator  logicop=AND  UseBitMask=on  BitMask=bin2dec('10000000')  BitMaskRealWorld=Stored Integer
  Bitwise Operator3 : simulink/Logic and Bit Operations/Bitwise Operator  logicop=AND  UseBitMask=on  BitMask=bin2dec('01111111')  BitMaskRealWorld=Stored Integer
  Constant4 : Constant  Value=127
  Constant5 : Constant  Value=8388608
  Constant7 : Constant  Value=-1
  Data Type Conversion : DataTypeConversion  OutDataTypeStr=uint8
  Data Type Conversion1 : DataTypeConversion  OutDataTypeStr=uint8
  Data Type Conversion{2..5} (4 alike) : DataTypeConversion  OutDataTypeStr=uint32
  Data Type Conversion7 : DataTypeConversion  OutDataTypeStr=double
  Display3 : Display
      settings: Format=binary (Stored Integer)
  Display4 : Display
      settings: Format=binary (Stored Integer)
  Exponent : Display
      settings: Format=binary (Stored Integer)
  Mantissa : Display
      settings: Format=binary (Stored Integer)
  Math Function : Math  Operator=pow  SaturateOnIntegerOverflow=on
  Product : Product  RndMeth=Zero
  Shift Arithmetic : simulink/Logic and Bit Operations/Shift Arithmetic  SystemSampleTime=-1  nBitShiftRight=-1  nBinPtShiftRight=0
  Shift Arithmetic1 : simulink/Logic and Bit Operations/Shift Arithmetic  SystemSampleTime=-1  nBitShiftRight=7  nBinPtShiftRight=0
  Shift Arithmetic2 : simulink/Logic and Bit Operations/Shift Arithmetic  SystemSampleTime=-1  nBitShiftRight=7  nBinPtShiftRight=0
  Shift Arithmetic3 : simulink/Logic and Bit Operations/Shift Arithmetic  SystemSampleTime=-1  nBitShiftRight=-16  nBinPtShiftRight=0
  Shift Arithmetic4 : simulink/Logic and Bit Operations/Shift Arithmetic  SystemSampleTime=-1  nBitShiftRight=-8  nBinPtShiftRight=0
  Sign : Display
      settings: Format=binary (Stored Integer)
  Subsystem : Subsystem
  Sum : Sum  Inputs=|++
  Sum1 : Sum  Inputs=|+++|
  Sum2 : Sum  Inputs=|+-
  Sum3 : Sum  Inputs=|++
  Out1 : Outport
  wires:
  Bitwise Operator/1 -> Display3/1, Shift Arithmetic/1
  Data Type Conversion/1 -> Bitwise Operator/1, Bitwise Operator2/1
  In2/1 -> Data Type Conversion2/1, Data Type Conversion1/1
  Data Type Conversion1/1 -> Bitwise Operator1/1
  Shift Arithmetic/1 -> Display4/1, Sum/1
  Bitwise Operator1/1 -> Shift Arithmetic1/1
  Shift Arithmetic1/1 -> Sum/2
  Sum/1 -> Exponent/1, Sum2/1
  Bitwise Operator2/1 -> Shift Arithmetic2/1
  Shift Arithmetic2/1 -> Sign/1, Data Type Conversion7/1
  Bitwise Operator3/1 -> Shift Arithmetic3/1
  Data Type Conversion2/1 -> Bitwise Operator3/1
  Shift Arithmetic3/1 -> Sum1/1
  Data Type Conversion3/1 -> Shift Arithmetic4/1
  Shift Arithmetic4/1 -> Sum1/2
  Data Type Conversion4/1 -> Sum1/3
  Sum1/1 -> Mantissa/1, Sum3/1
  Constant4/1 -> Sum2/2
  Sum2/1 -> Subsystem/1(In1)
  Sum3/1 -> Subsystem/2(In2)
  Constant5/1 -> Data Type Conversion5/1
  Data Type Conversion5/1 -> Sum3/2
  Subsystem/1(Out1) -> Product/2
  Constant7/1 -> Math Function/1
  Data Type Conversion7/1 -> Math Function/2
  Math Function/1 -> Product/1
  In1/1 -> Data Type Conversion/1
  Product/1 -> Out1/1
  In3/1 -> Data Type Conversion3/1
  In4/1 -> Data Type Conversion4/1

== system gnss_sdr_galileo_e1_tcp_connector_tracking_lib/gnss_sdr/gnss_sdr_galileo_e1_tcp_connector_tracking_rx/Subsystem10/hex2float ==
  In1 : Inport
  In2 : Inport  Port=2
  In3 : Inport  Port=3
  In4 : Inport  Port=4
  Bitwise Operator : simulink/Logic and Bit Operations/Bitwise Operator  logicop=AND  UseBitMask=on  BitMask=bin2dec('01111111')  BitMaskRealWorld=Stored Integer
  Bitwise Operator1 : simulink/Logic and Bit Operations/Bitwise Operator  logicop=AND  UseBitMask=on  BitMask=bin2dec('10000000')  BitMaskRealWorld=Stored Integer
  Bitwise Operator2 : simulink/Logic and Bit Operations/Bitwise Operator  logicop=AND  UseBitMask=on  BitMask=bin2dec('10000000')  BitMaskRealWorld=Stored Integer
  Bitwise Operator3 : simulink/Logic and Bit Operations/Bitwise Operator  logicop=AND  UseBitMask=on  BitMask=bin2dec('01111111')  BitMaskRealWorld=Stored Integer
  Constant4 : Constant  Value=127
  Constant5 : Constant  Value=8388608
  Constant7 : Constant  Value=-1
  Data Type Conversion : DataTypeConversion  OutDataTypeStr=uint8
  Data Type Conversion1 : DataTypeConversion  OutDataTypeStr=uint8
  Data Type Conversion{2..5} (4 alike) : DataTypeConversion  OutDataTypeStr=uint32
  Data Type Conversion7 : DataTypeConversion  OutDataTypeStr=double
  Display3 : Display
      settings: Format=binary (Stored Integer)
  Display4 : Display
      settings: Format=binary (Stored Integer)
  Exponent : Display
      settings: Format=binary (Stored Integer)
  Mantissa : Display
      settings: Format=binary (Stored Integer)
  Math Function : Math  Operator=pow  SaturateOnIntegerOverflow=on
  Product : Product  RndMeth=Zero
  Shift Arithmetic : simulink/Logic and Bit Operations/Shift Arithmetic  SystemSampleTime=-1  nBitShiftRight=-1  nBinPtShiftRight=0
  Shift Arithmetic1 : simulink/Logic and Bit Operations/Shift Arithmetic  SystemSampleTime=-1  nBitShiftRight=7  nBinPtShiftRight=0
  Shift Arithmetic2 : simulink/Logic and Bit Operations/Shift Arithmetic  SystemSampleTime=-1  nBitShiftRight=7  nBinPtShiftRight=0
  Shift Arithmetic3 : simulink/Logic and Bit Operations/Shift Arithmetic  SystemSampleTime=-1  nBitShiftRight=-16  nBinPtShiftRight=0
  Shift Arithmetic4 : simulink/Logic and Bit Operations/Shift Arithmetic  SystemSampleTime=-1  nBitShiftRight=-8  nBinPtShiftRight=0
  Sign : Display
      settings: Format=binary (Stored Integer)
  Subsystem : Subsystem
  Sum : Sum  Inputs=|++
  Sum1 : Sum  Inputs=|+++|
  Sum2 : Sum  Inputs=|+-
  Sum3 : Sum  Inputs=|++
  Out1 : Outport
  wires:
  Bitwise Operator/1 -> Display3/1, Shift Arithmetic/1
  Data Type Conversion/1 -> Bitwise Operator/1, Bitwise Operator2/1
  In2/1 -> Data Type Conversion2/1, Data Type Conversion1/1
  Data Type Conversion1/1 -> Bitwise Operator1/1
  Shift Arithmetic/1 -> Display4/1, Sum/1
  Bitwise Operator1/1 -> Shift Arithmetic1/1
  Shift Arithmetic1/1 -> Sum/2
  Sum/1 -> Exponent/1, Sum2/1
  Bitwise Operator2/1 -> Shift Arithmetic2/1
  Shift Arithmetic2/1 -> Sign/1, Data Type Conversion7/1
  Bitwise Operator3/1 -> Shift Arithmetic3/1
  Data Type Conversion2/1 -> Bitwise Operator3/1
  Shift Arithmetic3/1 -> Sum1/1
  Data Type Conversion3/1 -> Shift Arithmetic4/1
  Shift Arithmetic4/1 -> Sum1/2
  Data Type Conversion4/1 -> Sum1/3
  Sum1/1 -> Mantissa/1, Sum3/1
  Constant4/1 -> Sum2/2
  Sum2/1 -> Subsystem/1(In1)
  Sum3/1 -> Subsystem/2(In2)
  Constant5/1 -> Data Type Conversion5/1
  Data Type Conversion5/1 -> Sum3/2
  Subsystem/1(Out1) -> Product/2
  Constant7/1 -> Math Function/1
  Data Type Conversion7/1 -> Math Function/2
  Math Function/1 -> Product/1
  In1/1 -> Data Type Conversion/1
  Product/1 -> Out1/1
  In3/1 -> Data Type Conversion3/1
  In4/1 -> Data Type Conversion4/1

== system gnss_sdr_galileo_e1_tcp_connector_tracking_lib/gnss_sdr/gnss_sdr_galileo_e1_tcp_connector_tracking_rx/Subsystem11/hex2float ==
  In1 : Inport
  In2 : Inport  Port=2
  In3 : Inport  Port=3
  In4 : Inport  Port=4
  Bitwise Operator : simulink/Logic and Bit Operations/Bitwise Operator  logicop=AND  UseBitMask=on  BitMask=bin2dec('01111111')  BitMaskRealWorld=Stored Integer
  Bitwise Operator1 : simulink/Logic and Bit Operations/Bitwise Operator  logicop=AND  UseBitMask=on  BitMask=bin2dec('10000000')  BitMaskRealWorld=Stored Integer
  Bitwise Operator2 : simulink/Logic and Bit Operations/Bitwise Operator  logicop=AND  UseBitMask=on  BitMask=bin2dec('10000000')  BitMaskRealWorld=Stored Integer
  Bitwise Operator3 : simulink/Logic and Bit Operations/Bitwise Operator  logicop=AND  UseBitMask=on  BitMask=bin2dec('01111111')  BitMaskRealWorld=Stored Integer
  Constant4 : Constant  Value=127
  Constant5 : Constant  Value=8388608
  Constant7 : Constant  Value=-1
  Data Type Conversion : DataTypeConversion  OutDataTypeStr=uint8
  Data Type Conversion1 : DataTypeConversion  OutDataTypeStr=uint8
  Data Type Conversion{2..5} (4 alike) : DataTypeConversion  OutDataTypeStr=uint32
  Data Type Conversion7 : DataTypeConversion  OutDataTypeStr=double
  Display3 : Display
      settings: Format=binary (Stored Integer)
  Display4 : Display
      settings: Format=binary (Stored Integer)
  Exponent : Display
      settings: Format=binary (Stored Integer)
  Mantissa : Display
      settings: Format=binary (Stored Integer)
  Math Function : Math  Operator=pow  SaturateOnIntegerOverflow=on
  Product : Product  RndMeth=Zero
  Shift Arithmetic : simulink/Logic and Bit Operations/Shift Arithmetic  SystemSampleTime=-1  nBitShiftRight=-1  nBinPtShiftRight=0
  Shift Arithmetic1 : simulink/Logic and Bit Operations/Shift Arithmetic  SystemSampleTime=-1  nBitShiftRight=7  nBinPtShiftRight=0
  Shift Arithmetic2 : simulink/Logic and Bit Operations/Shift Arithmetic  SystemSampleTime=-1  nBitShiftRight=7  nBinPtShiftRight=0
  Shift Arithmetic3 : simulink/Logic and Bit Operations/Shift Arithmetic  SystemSampleTime=-1  nBitShiftRight=-16  nBinPtShiftRight=0
  Shift Arithmetic4 : simulink/Logic and Bit Operations/Shift Arithmetic  SystemSampleTime=-1  nBitShiftRight=-8  nBinPtShiftRight=0
  Sign : Display
      settings: Format=binary (Stored Integer)
  Subsystem : Subsystem
  Sum : Sum  Inputs=|++
  Sum1 : Sum  Inputs=|+++|
  Sum2 : Sum  Inputs=|+-
  Sum3 : Sum  Inputs=|++
  Out1 : Outport
  wires:
  In4/1 -> Data Type Conversion4/1
  In3/1 -> Data Type Conversion3/1
  Product/1 -> Out1/1
  In1/1 -> Data Type Conversion/1
  Math Function/1 -> Product/1
  Data Type Conversion7/1 -> Math Function/2
  Constant7/1 -> Math Function/1
  Subsystem/1(Out1) -> Product/2
  Data Type Conversion5/1 -> Sum3/2
  Constant5/1 -> Data Type Conversion5/1
  Sum3/1 -> Subsystem/2(In2)
  Sum2/1 -> Subsystem/1(In1)
  Constant4/1 -> Sum2/2
  Sum1/1 -> Sum3/1, Mantissa/1
  Data Type Conversion4/1 -> Sum1/3
  Shift Arithmetic4/1 -> Sum1/2
  Data Type Conversion3/1 -> Shift Arithmetic4/1
  Shift Arithmetic3/1 -> Sum1/1
  Data Type Conversion2/1 -> Bitwise Operator3/1
  Bitwise Operator3/1 -> Shift Arithmetic3/1
  Shift Arithmetic2/1 -> Data Type Conversion7/1, Sign/1
  Bitwise Operator2/1 -> Shift Arithmetic2/1
  Sum/1 -> Sum2/1, Exponent/1
  Shift Arithmetic1/1 -> Sum/2
  Bitwise Operator1/1 -> Shift Arithmetic1/1
  Shift Arithmetic/1 -> Sum/1, Display4/1
  Data Type Conversion1/1 -> Bitwise Operator1/1
  In2/1 -> Data Type Conversion1/1, Data Type Conversion2/1
  Data Type Conversion/1 -> Bitwise Operator2/1, Bitwise Operator/1
  Bitwise Operator/1 -> Shift Arithmetic/1, Display3/1

== system gnss_sdr_galileo_e1_tcp_connector_tracking_lib/gnss_sdr/gnss_sdr_galileo_e1_tcp_connector_tracking_rx/Subsystem12/hex2float ==
  In1 : Inport
  In2 : Inport  Port=2
  In3 : Inport  Port=3
  In4 : Inport  Port=4
  Bitwise Operator : simulink/Logic and Bit Operations/Bitwise Operator  logicop=AND  UseBitMask=on  BitMask=bin2dec('01111111')  BitMaskRealWorld=Stored Integer
  Bitwise Operator1 : simulink/Logic and Bit Operations/Bitwise Operator  logicop=AND  UseBitMask=on  BitMask=bin2dec('10000000')  BitMaskRealWorld=Stored Integer
  Bitwise Operator2 : simulink/Logic and Bit Operations/Bitwise Operator  logicop=AND  UseBitMask=on  BitMask=bin2dec('10000000')  BitMaskRealWorld=Stored Integer
  Bitwise Operator3 : simulink/Logic and Bit Operations/Bitwise Operator  logicop=AND  UseBitMask=on  BitMask=bin2dec('01111111')  BitMaskRealWorld=Stored Integer
  Constant4 : Constant  Value=127
  Constant5 : Constant  Value=8388608
  Constant7 : Constant  Value=-1
  Data Type Conversion : DataTypeConversion  OutDataTypeStr=uint8
  Data Type Conversion1 : DataTypeConversion  OutDataTypeStr=uint8
  Data Type Conversion{2..5} (4 alike) : DataTypeConversion  OutDataTypeStr=uint32
  Data Type Conversion7 : DataTypeConversion  OutDataTypeStr=double
  Display3 : Display
      settings: Format=binary (Stored Integer)
  Display4 : Display
      settings: Format=binary (Stored Integer)
  Exponent : Display
      settings: Format=binary (Stored Integer)
  Mantissa : Display
      settings: Format=binary (Stored Integer)
  Math Function : Math  Operator=pow  SaturateOnIntegerOverflow=on
  Product : Product  RndMeth=Zero
  Shift Arithmetic : simulink/Logic and Bit Operations/Shift Arithmetic  SystemSampleTime=-1  nBitShiftRight=-1  nBinPtShiftRight=0
  Shift Arithmetic1 : simulink/Logic and Bit Operations/Shift Arithmetic  SystemSampleTime=-1  nBitShiftRight=7  nBinPtShiftRight=0
  Shift Arithmetic2 : simulink/Logic and Bit Operations/Shift Arithmetic  SystemSampleTime=-1  nBitShiftRight=7  nBinPtShiftRight=0
  Shift Arithmetic3 : simulink/Logic and Bit Operations/Shift Arithmetic  SystemSampleTime=-1  nBitShiftRight=-16  nBinPtShiftRight=0
  Shift Arithmetic4 : simulink/Logic and Bit Operations/Shift Arithmetic  SystemSampleTime=-1  nBitShiftRight=-8  nBinPtShiftRight=0
  Sign : Display
      settings: Format=binary (Stored Integer)
  Subsystem : Subsystem
  Sum : Sum  Inputs=|++
  Sum1 : Sum  Inputs=|+++|
  Sum2 : Sum  Inputs=|+-
  Sum3 : Sum  Inputs=|++
  Out1 : Outport
  wires:
  Bitwise Operator/1 -> Display3/1, Shift Arithmetic/1
  Data Type Conversion/1 -> Bitwise Operator/1, Bitwise Operator2/1
  In2/1 -> Data Type Conversion2/1, Data Type Conversion1/1
  Data Type Conversion1/1 -> Bitwise Operator1/1
  Shift Arithmetic/1 -> Display4/1, Sum/1
  Bitwise Operator1/1 -> Shift Arithmetic1/1
  Shift Arithmetic1/1 -> Sum/2
  Sum/1 -> Exponent/1, Sum2/1
  Bitwise Operator2/1 -> Shift Arithmetic2/1
  Shift Arithmetic2/1 -> Sign/1, Data Type Conversion7/1
  Bitwise Operator3/1 -> Shift Arithmetic3/1
  Data Type Conversion2/1 -> Bitwise Operator3/1
  Shift Arithmetic3/1 -> Sum1/1
  Data Type Conversion3/1 -> Shift Arithmetic4/1
  Shift Arithmetic4/1 -> Sum1/2
  Data Type Conversion4/1 -> Sum1/3
  Sum1/1 -> Mantissa/1, Sum3/1
  Constant4/1 -> Sum2/2
  Sum2/1 -> Subsystem/1(In1)
  Sum3/1 -> Subsystem/2(In2)
  Constant5/1 -> Data Type Conversion5/1
  Data Type Conversion5/1 -> Sum3/2
  Subsystem/1(Out1) -> Product/2
  Constant7/1 -> Math Function/1
  Data Type Conversion7/1 -> Math Function/2
  Math Function/1 -> Product/1
  In1/1 -> Data Type Conversion/1
  Product/1 -> Out1/1
  In3/1 -> Data Type Conversion3/1
  In4/1 -> Data Type Conversion4/1
